simulink model "FLIGHT_Hexacopter_V2"  (R2025a)
settings: Solver=FixedStepDiscrete  StartTime=0.0  StopTime=inf  FixedStep=SampleTime_SAS  RelTol=1e-3  EnableMultiTasking=on
InitFcn:
  | Init_FLIGHT_Hexacopter
values from neighbouring files (symbols this model uses):
  d2r = pi/180    (= 0.0174532925199)    [Init_FLIGHT_Hexacopter.m]
  Kdrr = 0.004    [Init_FLIGHT_Hexacopter_fromNCMS.m]
  Kirr = 0.0    (= 0)    [Init_FLIGHT_Hexacopter_fromNCMS.m]
  Kpp = 3.3894    [Init_FLIGHT_Hexacopter_fromNCMS.m]
  Kpr = 3.3894    [Init_FLIGHT_Hexacopter_fromNCMS.m]
  Kprr = 0.1    [Init_FLIGHT_Hexacopter_fromNCMS.m]
  MAX_CONTROL_ANGLE_PITCH = 30*pi/180    (= 0.523598775598)    [Init_FLIGHT_Hexacopter.m]    (also in Init_FLIGHT_Hexacopter_fromNCMS.m = 0.349065850399)
  MAX_CONTROL_ANGLE_RATE_PITCH = 360*pi/180    (= 6.28318530718)    [Init_FLIGHT_Hexacopter.m]    (also in Init_FLIGHT_Hexacopter_fromNCMS.m)
  MAX_CONTROL_ANGLE_RATE_ROLL = 360*pi/180    (= 6.28318530718)    [Init_FLIGHT_Hexacopter.m]    (also in Init_FLIGHT_Hexacopter_fromNCMS.m)
  MAX_CONTROL_ANGLE_RATE_Y = 120*pi/180    (= 2.09439510239)    [Init_FLIGHT_Hexacopter.m]    (also in Init_FLIGHT_Hexacopter_fromNCMS.m)
  MAX_CONTROL_ANGLE_ROLL = 30*pi/180    (= 0.523598775598)    [Init_FLIGHT_Hexacopter.m]    (also in Init_FLIGHT_Hexacopter_fromNCMS.m = 0.349065850399)
  Nrr = 50    [Init_FLIGHT_Hexacopter_fromNCMS.m]
  PITCH_AUTHORITY = 1    [Init_FLIGHT_Hexacopter.m]
  ROLL_AUTHORITY = 1    [Init_FLIGHT_Hexacopter.m]
  SampleTime = 1/250    (= 0.004)    [Init_FLIGHT_Hexacopter.m]    (also in Init_FLIGHT_Hexacopter_fromNCMS.m = 0.01)
  SampleTime_SAS = 1/1000    (= 0.001)    [Init_FLIGHT_Hexacopter.m]
  YAW_AUTHORITY = 1    [Init_FLIGHT_Hexacopter.m]
undefined symbols (not defined in the file or in its folder): arguments, DiscIntNeverNeededParam, e_dot, event_sequence, fx, g1x, hx, id, integral_e, log_levels, MPC_Z_D, MPC_Z_I, MPC_Z_P, noutputs, omega, omega_dot, output, phi_cmd, phi_cmd_ddot, phi_cmd_dot, r, s, tau_roll, timestamp, w
libraries: px4Utilslib x65, simulink x21, px4uORBlib x12, slpidlib x9, cstblocks x5, simulink_extras x2, sharedtransform x1, px4Sensorslib x1, matrix_library x1, px4Peripheralslib x1
(part 2 of 3)

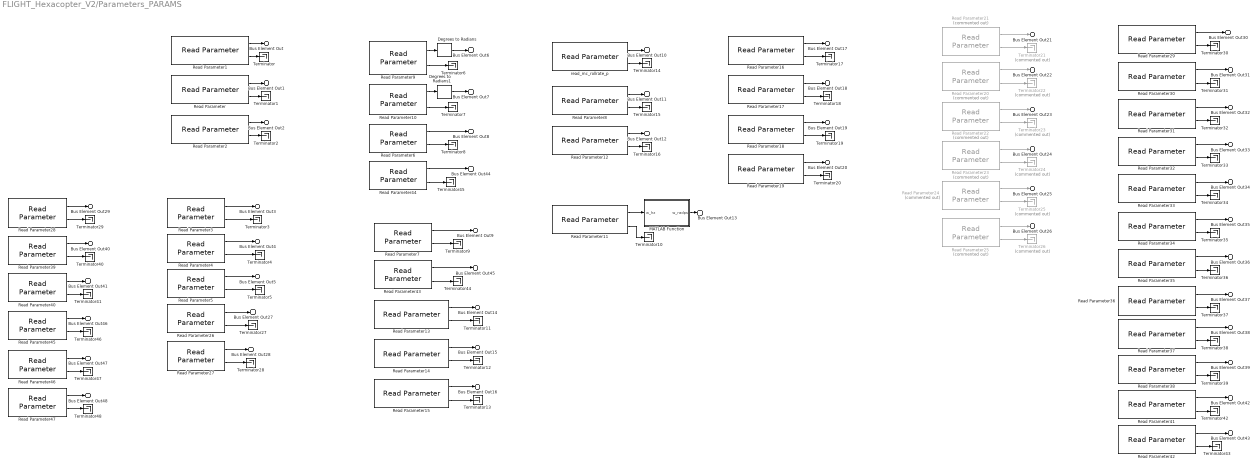
== system FLIGHT_Hexacopter_V2/Parameters_PARAMS ==
  Degrees to Radians : simulink_extras/Transformations/Degrees to Radians
  Degrees to Radians1 : simulink_extras/Transformations/Degrees to Radians
  MATLAB Function : MATLAB Function  TreatAsAtomicUnit=on
  Read Parameter : px4Utilslib/Read Parameter  ParameterName=DOUBLET_DT  DataType=FLOAT  SampleTime=SampleTime
  Read Parameter1 : px4Utilslib/Read Parameter  ParameterName=DOUBLET_PEAK_ANG  DataType=FLOAT  SampleTime=SampleTime
  Read Parameter10 : px4Utilslib/Read Parameter  ParameterName=MC_PITCHRATE_MAX  DataType=FLOAT  SampleTime=SampleTime
  Read Parameter11 : px4Utilslib/Read Parameter  ParameterName=IMU_DGYRO_CUTOFF  DataType=FLOAT  SampleTime=SampleTime
  Read Parameter12 : px4Utilslib/Read Parameter  ParameterName=MC_ROLLRATE_D  DataType=FLOAT  SampleTime=SampleTime
  Read Parameter13 : px4Utilslib/Read Parameter  ParameterName=MC_PITCHRATE_P  DataType=FLOAT  SampleTime=SampleTime
  Read Parameter14 : px4Utilslib/Read Parameter  ParameterName=MC_PITCHRATE_I  DataType=FLOAT  SampleTime=SampleTime
  Read Parameter15 : px4Utilslib/Read Parameter  ParameterName=MC_PITCHRATE_D  DataType=FLOAT  SampleTime=SampleTime
  Read Parameter16 : px4Utilslib/Read Parameter  ParameterName=MC_YAWRATE_P  DataType=FLOAT  SampleTime=SampleTime
  Read Parameter17 : px4Utilslib/Read Parameter  ParameterName=MC_YAWRATE_I  DataType=FLOAT  SampleTime=SampleTime
  Read Parameter18 : px4Utilslib/Read Parameter  ParameterName=MC_YAWRATE_D  DataType=FLOAT  SampleTime=SampleTime
  Read Parameter19 : px4Utilslib/Read Parameter  ParameterName=MC_YAWRATE_FF  DataType=FLOAT  SampleTime=SampleTime
  Read Parameter2 : px4Utilslib/Read Parameter  ParameterName=DOUBLET_AXIS  DataType=INT32  SampleTime=SampleTime
  Read Parameter20 : px4Utilslib/Read Parameter  Commented=on  ParameterName=FDD_M2_STATUS  DataType=INT32  SampleTime=SampleTime
  Read Parameter21 : px4Utilslib/Read Parameter  Commented=on  ParameterName=FDD_M1_STATUS  DataType=INT32  SampleTime=SampleTime
  Read Parameter22 : px4Utilslib/Read Parameter  Commented=on  ParameterName=FDD_M3_STATUS  DataType=INT32  SampleTime=SampleTime
  Read Parameter23 : px4Utilslib/Read Parameter  Commented=on  ParameterName=FDD_M4_STATUS  DataType=INT32  SampleTime=SampleTime
  Read Parameter24 : px4Utilslib/Read Parameter  Commented=on  ParameterName=FDD_M5_STATUS  DataType=INT32  SampleTime=SampleTime
  Read Parameter25 : px4Utilslib/Read Parameter  Commented=on  ParameterName=FDD_M6_STATUS  DataType=INT32  SampleTime=SampleTime
  Read Parameter26 : px4Utilslib/Read Parameter  ParameterName=MPC_THR_HOVER  DataType=FLOAT  SampleTime=SampleTime
  Read Parameter27 : px4Utilslib/Read Parameter  ParameterName=MPC_XY_P  DataType=FLOAT  SampleTime=SampleTime
  Read Parameter28 : px4Utilslib/Read Parameter  ParameterName=MPC_XY_VEL_P_ACC  DataType=FLOAT  SampleTime=SampleTime
  Read Parameter29 : px4Utilslib/Read Parameter  ParameterName=SMC_K_SS_P  DataType=FLOAT  SampleTime=SampleTime
  Read Parameter3 : px4Utilslib/Read Parameter  ParameterName=MPC_Z_VEL_P_ACC  DataType=FLOAT  SampleTime=SampleTime
  Read Parameter30 : px4Utilslib/Read Parameter  ParameterName=SMC_K_SS_I  DataType=FLOAT  SampleTime=SampleTime
  Read Parameter31 : px4Utilslib/Read Parameter  ParameterName=SMC_K_SS_D  DataType=FLOAT  SampleTime=SampleTime
  Read Parameter32 : px4Utilslib/Read Parameter  ParameterName=SMC_K_REACH_S  DataType=FLOAT  SampleTime=SampleTime
  Read Parameter33 : px4Utilslib/Read Parameter  ParameterName=SMC_K_REACH_P  DataType=FLOAT  SampleTime=SampleTime
  Read Parameter34 : px4Utilslib/Read Parameter  ParameterName=SMC_I_XX  DataType=FLOAT  SampleTime=SampleTime
  Read Parameter35 : px4Utilslib/Read Parameter  ParameterName=SMC_I_YY  DataType=FLOAT  SampleTime=SampleTime
  Read Parameter36 : px4Utilslib/Read Parameter  ParameterName=SMC_I_ZZ  DataType=FLOAT  SampleTime=SampleTime
  Read Parameter37 : px4Utilslib/Read Parameter  ParameterName=SMC_EPSILON  DataType=FLOAT  SampleTime=SampleTime
  Read Parameter38 : px4Utilslib/Read Parameter  ParameterName=SMC_LPF_CUTOFF  DataType=FLOAT  SampleTime=SampleTime
  Read Parameter39 : px4Utilslib/Read Parameter  ParameterName=MPC_Z_VEL_MAX_UP  DataType=FLOAT  SampleTime=SampleTime
  Read Parameter4 : px4Utilslib/Read Parameter  ParameterName=MPC_Z_VEL_I_ACC  DataType=FLOAT  SampleTime=SampleTime
  Read Parameter40 : px4Utilslib/Read Parameter  ParameterName=MPC_XY_VEL_MAX  DataType=FLOAT  SampleTime=SampleTime
  Read Parameter41 : px4Utilslib/Read Parameter  ParameterName=ST_SMC_LAMBDA  DataType=FLOAT  SampleTime=SampleTime
  Read Parameter42 : px4Utilslib/Read Parameter  ParameterName=ST_SMC_ETA  DataType=FLOAT  SampleTime=SampleTime
  Read Parameter43 : px4Utilslib/Read Parameter  ParameterName=MC_PITCH_I  DataType=FLOAT  SampleTime=SampleTime
  Read Parameter44 : px4Utilslib/Read Parameter  ParameterName=MC_ROLL_I  DataType=FLOAT  SampleTime=SampleTime
  Read Parameter45 : px4Utilslib/Read Parameter  ParameterName=MPC_XY_VEL_I_ACC  DataType=FLOAT  SampleTime=SampleTime
  Read Parameter46 : px4Utilslib/Read Parameter  ParameterName=MPC_XY_VEL_D_ACC  DataType=FLOAT  SampleTime=SampleTime
  Read Parameter47 : px4Utilslib/Read Parameter  ParameterName=MPC_WP_LENGTH  DataType=FLOAT  SampleTime=SampleTime
  Read Parameter5 : px4Utilslib/Read Parameter  ParameterName=MPC_Z_VEL_D_ACC  DataType=FLOAT  SampleTime=SampleTime
  Read Parameter6 : px4Utilslib/Read Parameter  ParameterName=MC_ROLL_P  DataType=FLOAT  SampleTime=SampleTime
  Read Parameter7 : px4Utilslib/Read Parameter  ParameterName=MC_PITCH_P  DataType=FLOAT  SampleTime=SampleTime
  Read Parameter8 : px4Utilslib/Read Parameter  ParameterName=MC_ROLLRATE_I  DataType=FLOAT  SampleTime=SampleTime
  Read Parameter9 : px4Utilslib/Read Parameter  ParameterName=MC_ROLLRATE_MAX  DataType=FLOAT  SampleTime=SampleTime
  Terminator{,1..20,27..48} (43 alike) : Terminator
  Terminator{21..26} (6 alike) : Terminator  Commented=on
  read_mc_rollrate_p : px4Utilslib/Read Parameter  ParameterName=MC_ROLLRATE_P  DataType=FLOAT  SampleTime=SampleTime
  Bus Element Out : Outport  PortName=PARAMS  Element=DOUBLET_PEAK_ANG
  Bus Element Out1 : Outport  PortName=PARAMS  Element=DOUBLET_DT
  Bus Element Out2 : Outport  PortName=PARAMS  Element=DOUBLET_AXIS
  Bus Element Out3 : Outport  PortName=PARAMS  Element=MPC_Z_VEL_P_ACC
  Bus Element Out4 : Outport  PortName=PARAMS  Element=MPC_Z_VEL_I_ACC
  Bus Element Out5 : Outport  PortName=PARAMS  Element=MPC_Z_VEL_D_ACC
  Bus Element Out6 : Outport  PortName=PARAMS  Element=MC_ROLLRATE_MAX
  Bus Element Out7 : Outport  PortName=PARAMS  Element=MC_PITCHRATE_MAX
  Bus Element Out8 : Outport  PortName=PARAMS  Element=MC_ROLL_P
  Bus Element Out9 : Outport  PortName=PARAMS  Element=MC_PITCH_P
  Bus Element Out10 : Outport  PortName=PARAMS  Element=MC_ROLLRATE_P
  Bus Element Out11 : Outport  PortName=PARAMS  Element=MC_ROLLRATE_I
  Bus Element Out12 : Outport  PortName=PARAMS  Element=MC_ROLLRATE_D
  Bus Element Out13 : Outport  PortName=PARAMS  Element=IMU_DGYRO_CUTOFF
  Bus Element Out14 : Outport  PortName=PARAMS  Element=MC_PITCHRATE_P
  Bus Element Out15 : Outport  PortName=PARAMS  Element=MC_PITCHRATE_I
  Bus Element Out16 : Outport  PortName=PARAMS  Element=MC_PITCHRATE_D
  Bus Element Out17 : Outport  PortName=PARAMS  Element=MC_YAWRATE_P
  Bus Element Out18 : Outport  PortName=PARAMS  Element=MC_YAWRATE_I
  Bus Element Out19 : Outport  PortName=PARAMS  Element=MC_YAWRATE_D
  Bus Element Out20 : Outport  PortName=PARAMS  Element=MC_YAWRATE_FF
  Bus Element Out21 : Outport  PortName=PARAMS  Element=FDD_M1_STATUS
  Bus Element Out22 : Outport  PortName=PARAMS  Element=FDD_M2_STATUS
  Bus Element Out23 : Outport  PortName=PARAMS  Element=FDD_M3_STATUS
  Bus Element Out24 : Outport  PortName=PARAMS  Element=FDD_M4_STATUS
  Bus Element Out25 : Outport  PortName=PARAMS  Element=FDD_M5_STATUS
  Bus Element Out26 : Outport  PortName=PARAMS  Element=FDD_M6_STATUS
  Bus Element Out27 : Outport  PortName=PARAMS  Element=MPC_THR_HOVER
  Bus Element Out28 : Outport  PortName=PARAMS  Element=MPC_XY_P
  Bus Element Out29 : Outport  PortName=PARAMS  Element=MPC_XY_VEL_P_ACC
  Bus Element Out30 : Outport  PortName=PARAMS  Element=K_SMC_P
  Bus Element Out31 : Outport  PortName=PARAMS  Element=K_SMC_I
  Bus Element Out32 : Outport  PortName=PARAMS  Element=K_SMC_D
  Bus Element Out33 : Outport  PortName=PARAMS  Element=K_REACH_S
  Bus Element Out34 : Outport  PortName=PARAMS  Element=K_REACH_P
  Bus Element Out35 : Outport  PortName=PARAMS  Element=I_XX
  Bus Element Out36 : Outport  PortName=PARAMS  Element=I_YY
  Bus Element Out37 : Outport  PortName=PARAMS  Element=I_ZZ
  Bus Element Out38 : Outport  PortName=PARAMS  Element=EPSILON
  Bus Element Out39 : Outport  PortName=PARAMS  Element=SMC_LPF_CUTOFF
  Bus Element Out40 : Outport  PortName=PARAMS  Element=MPC_Z_VEL_MAX_UP
  Bus Element Out41 : Outport  PortName=PARAMS  Element=MPC_XY_VEL_MAX
  Bus Element Out42 : Outport  PortName=PARAMS  Element=ST_SMC_LAMBDA
  Bus Element Out43 : Outport  PortName=PARAMS  Element=ST_SMC_ETA
  Bus Element Out44 : Outport  PortName=PARAMS  Element=MC_ROLL_I
  Bus Element Out45 : Outport  PortName=PARAMS  Element=MC_PITCH_I
  Bus Element Out46 : Outport  PortName=PARAMS  Element=MPC_XY_VEL_I_ACC
  Bus Element Out47 : Outport  PortName=PARAMS  Element=MPC_XY_VEL_D_ACC
  Bus Element Out48 : Outport  PortName=PARAMS  Element=MPC_WP_LENGTH
  wires:
  Read Parameter9/2 -> Terminator6/1
  Read Parameter10/1 -> Degrees to Radians1/1
  Read Parameter9/1 -> Degrees to Radians/1
  Read Parameter10/2 -> Terminator7/1
  Read Parameter7/1 -> Bus Element Out9/1
  Read Parameter7/2 -> Terminator9/1
  Read Parameter6/1 -> Bus Element Out8/1
  Read Parameter6/2 -> Terminator8/1
  Read Parameter11/2 -> Terminator10/1
  Read Parameter11/1 -> MATLAB Function/1(w_hz)
  Read Parameter1/1 -> Bus Element Out/1
  Read Parameter1/2 -> Terminator/1
  Read Parameter2/1 -> Bus Element Out2/1
  Read Parameter2/2 -> Terminator2/1
  Read Parameter/2 -> Terminator1/1
  Read Parameter/1 -> Bus Element Out1/1
  Read Parameter3/1 -> Bus Element Out3/1
  Read Parameter4/1 -> Bus Element Out4/1
  Read Parameter5/1 -> Bus Element Out5/1
  Read Parameter3/2 -> Terminator3/1
  Read Parameter4/2 -> Terminator4/1
  Read Parameter5/2 -> Terminator5/1
  Degrees to Radians1/1 -> Bus Element Out7/1
  Degrees to Radians/1 -> Bus Element Out6/1
  read_mc_rollrate_p/1 -> Bus Element Out10/1
  Read Parameter8/1 -> Bus Element Out11/1
  Read Parameter12/1 -> Bus Element Out12/1
  MATLAB Function/1(w_radps) -> Bus Element Out13/1
  Read Parameter13/1 -> Bus Element Out14/1
  Read Parameter14/1 -> Bus Element Out15/1
  Read Parameter15/1 -> Bus Element Out16/1
  Read Parameter13/2 -> Terminator11/1
  Read Parameter14/2 -> Terminator12/1
  Read Parameter15/2 -> Terminator13/1
  read_mc_rollrate_p/2 -> Terminator14/1
  Read Parameter8/2 -> Terminator15/1
  Read Parameter12/2 -> Terminator16/1
  Read Parameter16/1 -> Bus Element Out17/1
  Read Parameter17/1 -> Bus Element Out18/1
  Read Parameter18/1 -> Bus Element Out19/1
  Read Parameter19/1 -> Bus Element Out20/1
  Read Parameter16/2 -> Terminator17/1
  Read Parameter17/2 -> Terminator18/1
  Read Parameter18/2 -> Terminator19/1
  Read Parameter19/2 -> Terminator20/1
  Read Parameter21/1 -> Bus Element Out21/1
  Read Parameter20/1 -> Bus Element Out22/1
  Read Parameter22/1 -> Bus Element Out23/1
  Read Parameter23/1 -> Bus Element Out24/1
  Read Parameter24/1 -> Bus Element Out25/1
  Read Parameter25/1 -> Bus Element Out26/1
  Read Parameter21/2 -> Terminator21/1
  Read Parameter20/2 -> Terminator22/1
  Read Parameter22/2 -> Terminator23/1
  Read Parameter23/2 -> Terminator24/1
  Read Parameter24/2 -> Terminator25/1
  Read Parameter25/2 -> Terminator26/1
  Read Parameter26/1 -> Bus Element Out27/1
  Read Parameter26/2 -> Terminator27/1
  Read Parameter27/1 -> Bus Element Out28/1
  Read Parameter27/2 -> Terminator28/1
  Read Parameter28/1 -> Bus Element Out29/1
  Read Parameter28/2 -> Terminator29/1
  Read Parameter32/1 -> Bus Element Out33/1
  Read Parameter33/2 -> Terminator34/1
  Read Parameter31/2 -> Terminator32/1
  Read Parameter33/1 -> Bus Element Out34/1
  Read Parameter29/1 -> Bus Element Out30/1
  Read Parameter30/2 -> Terminator31/1
  Read Parameter30/1 -> Bus Element Out31/1
  Read Parameter32/2 -> Terminator33/1
  Read Parameter31/1 -> Bus Element Out32/1
  Read Parameter29/2 -> Terminator30/1
  Read Parameter34/1 -> Bus Element Out35/1
  Read Parameter34/2 -> Terminator35/1
  Read Parameter35/1 -> Bus Element Out36/1
  Read Parameter35/2 -> Terminator36/1
  Read Parameter36/1 -> Bus Element Out37/1
  Read Parameter36/2 -> Terminator37/1
  Read Parameter37/1 -> Bus Element Out38/1
  Read Parameter37/2 -> Terminator38/1
  Read Parameter38/1 -> Bus Element Out39/1
  Read Parameter38/2 -> Terminator39/1
  Read Parameter39/2 -> Terminator40/1
  Read Parameter39/1 -> Bus Element Out40/1
  Read Parameter40/1 -> Bus Element Out41/1
  Read Parameter40/2 -> Terminator41/1
  Read Parameter41/1 -> Bus Element Out42/1
  Read Parameter41/2 -> Terminator42/1
  Read Parameter42/1 -> Bus Element Out43/1
  Read Parameter42/2 -> Terminator43/1
  Read Parameter43/1 -> Bus Element Out45/1
  Read Parameter43/2 -> Terminator44/1
  Read Parameter44/1 -> Bus Element Out44/1
  Read Parameter44/2 -> Terminator45/1
  Read Parameter45/1 -> Bus Element Out46/1
  Read Parameter46/1 -> Bus Element Out47/1
  Read Parameter45/2 -> Terminator46/1
  Read Parameter46/2 -> Terminator47/1
  Read Parameter47/1 -> Bus Element Out48/1
  Read Parameter47/2 -> Terminator48/1

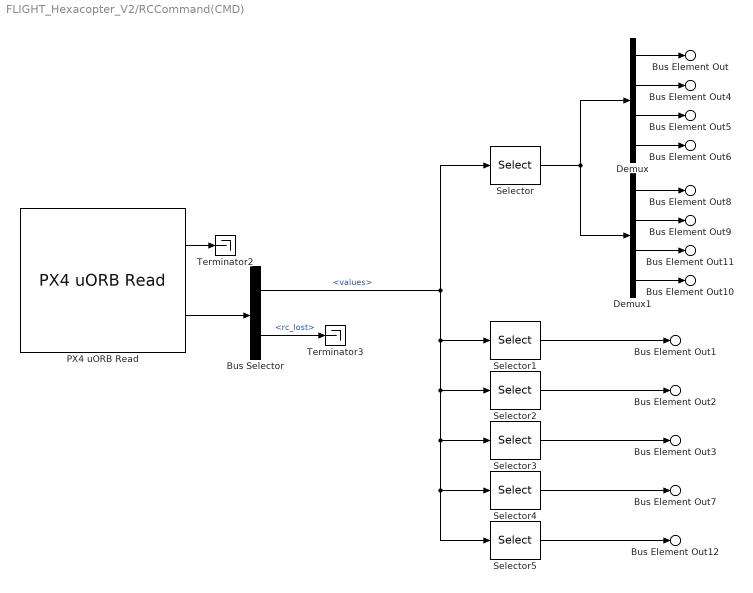
== system FLIGHT_Hexacopter_V2/RCCommand(CMD) ==
  Bus Selector : BusSelector  OutputSignals=values,rc_lost
  Demux : Demux
  Demux1 : Demux
  PX4 uORB Read : px4uORBlib/PX4 uORB Read  uORBTopic=InputRc  selectInstance=InputRc  SampleTime=SampleTime  BlockingMode=off  BlockTimeout=1e-3
  Selector : Selector  InputPortWidth=18  IndexOptions=Index vector (dialog)  Indices=[1 2 4 3]  OutputSizes=1
  Selector1 : Selector  InputPortWidth=18  IndexOptions=Index vector (dialog)  Indices=[6]  OutputSizes=1
  Selector2 : Selector  InputPortWidth=18  IndexOptions=Index vector (dialog)  Indices=7  OutputSizes=1
  Selector3 : Selector  InputPortWidth=18  IndexOptions=Index vector (dialog)  Indices=8  OutputSizes=1
  Selector4 : Selector  InputPortWidth=18  IndexOptions=Index vector (dialog)  Indices=10  OutputSizes=1
  Selector5 : Selector  InputPortWidth=18  IndexOptions=Index vector (dialog)  Indices=11  OutputSizes=1
  Terminator2 : Terminator
  Terminator3 : Terminator
  Bus Element Out : Outport  PortName=CMD  Element=rc_mode2_roll
  Bus Element Out1 : Outport  PortName=CMD  Element=rc_mode
  Bus Element Out2 : Outport  PortName=CMD  Element=rc_doublet
  Bus Element Out3 : Outport  PortName=CMD  Element=rc_inject_failure
  Bus Element Out4 : Outport  PortName=CMD  Element=rc_mode2_pitch
  Bus Element Out5 : Outport  PortName=CMD  Element=rc_mode2_yaw
  Bus Element Out6 : Outport  PortName=CMD  Element=rc_mode2_throttle
  Bus Element Out7 : Outport  PortName=CMD  Element=rc_ctrl_switch
  Bus Element Out8 : Outport  PortName=CMD  Element=rc_mode1_roll
  Bus Element Out9 : Outport  PortName=CMD  Element=rc_mode1_throttle
  Bus Element Out10 : Outport  PortName=CMD  Element=rc_mode1_pitch
  Bus Element Out11 : Outport  PortName=CMD  Element=rc_mode1_yaw
  Bus Element Out12 : Outport  PortName=CMD  Element=rc_ap_sw
  wires:
  Selector/1 -> Demux1/1, Demux/1
  PX4 uORB Read/2 -> Bus Selector/1
  Bus Selector/2 -> Terminator3/1  "<rc_lost>"
  Selector1/1 -> Bus Element Out1/1
  Bus Selector/1 -> Selector5/1, Selector4/1, Selector3/1, Selector2/1, Selector1/1, Selector/1  "<values>"
  PX4 uORB Read/1 -> Terminator2/1
  Demux/1 -> Bus Element Out/1
  Demux/2 -> Bus Element Out4/1
  Demux/3 -> Bus Element Out5/1
  Demux/4 -> Bus Element Out6/1
  Selector2/1 -> Bus Element Out2/1
  Selector3/1 -> Bus Element Out3/1
  Selector4/1 -> Bus Element Out7/1
  Demux1/1 -> Bus Element Out8/1
  Demux1/2 -> Bus Element Out9/1
  Demux1/3 -> Bus Element Out11/1
  Demux1/4 -> Bus Element Out10/1
  Selector5/1 -> Bus Element Out12/1

== system FLIGHT_Hexacopter_V2/Read_uORB(1000hz)_SENSORS1000 ==
  Bus Selector2 : BusSelector  OutputSignals=xyz,xyz_derivative
  Demux : Demux  Outputs=3
  Demux1 : Demux  Outputs=3
  PX4 uORB Read1 : px4uORBlib/PX4 uORB Read  uORBTopic=VehicleAngularVelocity  selectInstance=vehicle_angular_velocity  SampleTime=SampleTime_SAS  BlockingMode=off  BlockTimeout=1e-3
  Terminator1 : Terminator
  Bus Element Out : Outport  PortName=SENSORS1000  Element=P
  Bus Element Out1 : Outport  PortName=SENSORS1000  Element=Q
  Bus Element Out2 : Outport  PortName=SENSORS1000  Element=R
  Bus Element Out3 : Outport  PortName=SENSORS1000  Element=P_dot
  Bus Element Out4 : Outport  PortName=SENSORS1000  Element=Q_dot
  Bus Element Out5 : Outport  PortName=SENSORS1000  Element=R_dot
  wires:
  Bus Selector2/1 -> Demux/1  "<xyz>"
  PX4 uORB Read1/1 -> Terminator1/1
  Bus Selector2/2 -> Demux1/1  "<xyz_derivative>"
  PX4 uORB Read1/2 -> Bus Selector2/1
  Demux/1 -> Bus Element Out/1
  Demux/2 -> Bus Element Out1/1
  Demux/3 -> Bus Element Out2/1
  Demux1/1 -> Bus Element Out3/1
  Demux1/2 -> Bus Element Out4/1
  Demux1/3 -> Bus Element Out5/1

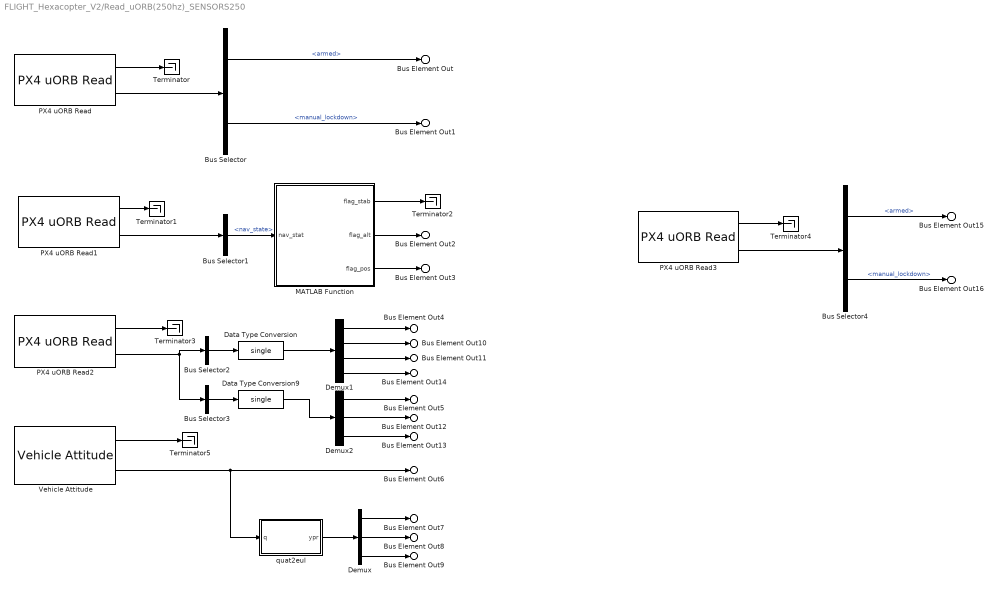
== system FLIGHT_Hexacopter_V2/Read_uORB(250hz)_SENSORS250 ==
  Bus Selector : BusSelector  OutputSignals=armed,manual_lockdown
  Bus Selector1 : BusSelector  OutputSignals=nav_state
  Bus Selector2 : BusSelector  OutputSignals=x,y,z,heading  OutputAsBus=on
  Bus Selector3 : BusSelector  OutputSignals=vx,vy,vz  OutputAsBus=on
  Bus Selector4 : BusSelector  OutputSignals=armed,manual_lockdown
  Data Type Conversion : DataTypeConversion  OutDataTypeStr=single  SaturateOnIntegerOverflow=off  RndMeth=Floor
  Data Type Conversion9 : DataTypeConversion  OutDataTypeStr=single  SaturateOnIntegerOverflow=off  RndMeth=Floor
  Demux : Demux  Outputs=3
  Demux1 : Demux
  Demux2 : Demux  Outputs=3
  MATLAB Function : MATLAB Function  TreatAsAtomicUnit=on
  PX4 uORB Read : px4uORBlib/PX4 uORB Read  uORBTopic=ActuatorArmed  selectInstance=ActuatorArmed  SampleTime=SampleTime  BlockingMode=off  BlockTimeout=1e-3
  PX4 uORB Read1 : px4uORBlib/PX4 uORB Read  uORBTopic=VehicleStatus  selectInstance=VehicleStatus  SampleTime=SampleTime  BlockingMode=off  BlockTimeout=1e-3
  PX4 uORB Read2 : px4uORBlib/PX4 uORB Read  uORBTopic=VehicleLocalPosition  selectInstance=vehicle_local_position  SampleTime=SampleTime  BlockingMode=off  BlockTimeout=1e-3
  PX4 uORB Read3 : px4uORBlib/PX4 uORB Read  uORBTopic=ActuatorArmed  selectInstance=ActuatorArmed  SampleTime=SampleTime  BlockingMode=off  BlockTimeout=1e-3
  Terminator{,1..5} (6 alike) : Terminator
  Vehicle Attitude : px4Sensorslib/Vehicle Attitude  rollRate=off  pitchRate=off  yawRate=off  quaternion=on  uorbTimeStamp=off  BlockingMode=off  BlockTimeout=0.001  sampleTime=SampleTime
  quat2eul : MATLAB Function  TreatAsAtomicUnit=on
  Bus Element Out : Outport  PortName=SENSORS250  Element=VehicleStatus_armed
  Bus Element Out1 : Outport  PortName=SENSORS250  Element=VehicleStatus_emergency_kill
  Bus Element Out2 : Outport  PortName=SENSORS250  Element=VehicleStatus_flag_altitude_mode
  Bus Element Out3 : Outport  PortName=SENSORS250  Element=VehicleStatus_flag_position_mode
  Bus Element Out4 : Outport  PortName=SENSORS250  Element=X
  Bus Element Out5 : Outport  PortName=SENSORS250  Element=U
  Bus Element Out6 : Outport  PortName=SENSORS250  Element=State_quaternion
  Bus Element Out7 : Outport  PortName=SENSORS250  Element=Psi
  Bus Element Out8 : Outport  PortName=SENSORS250  Element=Theta
  Bus Element Out9 : Outport  PortName=SENSORS250  Element=Phi
  Bus Element Out12 : Outport  PortName=SENSORS250  Element=V
  Bus Element Out13 : Outport  PortName=SENSORS250  Element=W
  Bus Element Out10 : Outport  PortName=SENSORS250  Element=Y
  Bus Element Out11 : Outport  PortName=SENSORS250  Element=Z
  Bus Element Out14 : Outport  PortName=SENSORS250  Element=Heading
  Bus Element Out15 : Outport  PortName=SENSORS250  Element=VehicleStatus_flag_armed
  Bus Element Out16 : Outport  PortName=SENSORS250  Element=VehicleStatus_flag_kill
  wires:
  Bus Selector/2 -> Bus Element Out1/1  "<manual_lockdown>"
  Bus Selector/1 -> Bus Element Out/1  "<armed>"
  PX4 uORB Read/1 -> Terminator/1
  PX4 uORB Read/2 -> Bus Selector/1
  PX4 uORB Read1/1 -> Terminator1/1
  PX4 uORB Read1/2 -> Bus Selector1/1
  MATLAB Function/3(flag_pos) -> Bus Element Out3/1
  Bus Selector1/1 -> MATLAB Function/1(nav_stat)  "<nav_state>"
  MATLAB Function/2(flag_alt) -> Bus Element Out2/1
  MATLAB Function/1(flag_stab) -> Terminator2/1
  Bus Selector3/1 -> Data Type Conversion9/1
  PX4 uORB Read2/1 -> Terminator3/1
  Bus Selector2/1 -> Data Type Conversion/1
  Vehicle Attitude/1 -> Terminator5/1
  PX4 uORB Read2/2 -> Bus Selector3/1, Bus Selector2/1
  Vehicle Attitude/2 -> quat2eul/1(q), Bus Element Out6/1
  quat2eul/1(ypr) -> Demux/1
  Demux/1 -> Bus Element Out7/1
  Demux/2 -> Bus Element Out8/1
  Demux/3 -> Bus Element Out9/1
  Data Type Conversion/1 -> Demux1/1
  Demux1/1 -> Bus Element Out4/1
  Demux1/2 -> Bus Element Out10/1
  Demux1/3 -> Bus Element Out11/1
  Data Type Conversion9/1 -> Demux2/1
  Demux2/1 -> Bus Element Out5/1
  Demux2/2 -> Bus Element Out12/1
  Demux2/3 -> Bus Element Out13/1
  Demux1/4 -> Bus Element Out14/1
  PX4 uORB Read3/2 -> Bus Selector4/1
  PX4 uORB Read3/1 -> Terminator4/1
  Bus Selector4/2 -> Bus Element Out16/1  "<manual_lockdown>"
  Bus Selector4/1 -> Bus Element Out15/1  "<armed>"

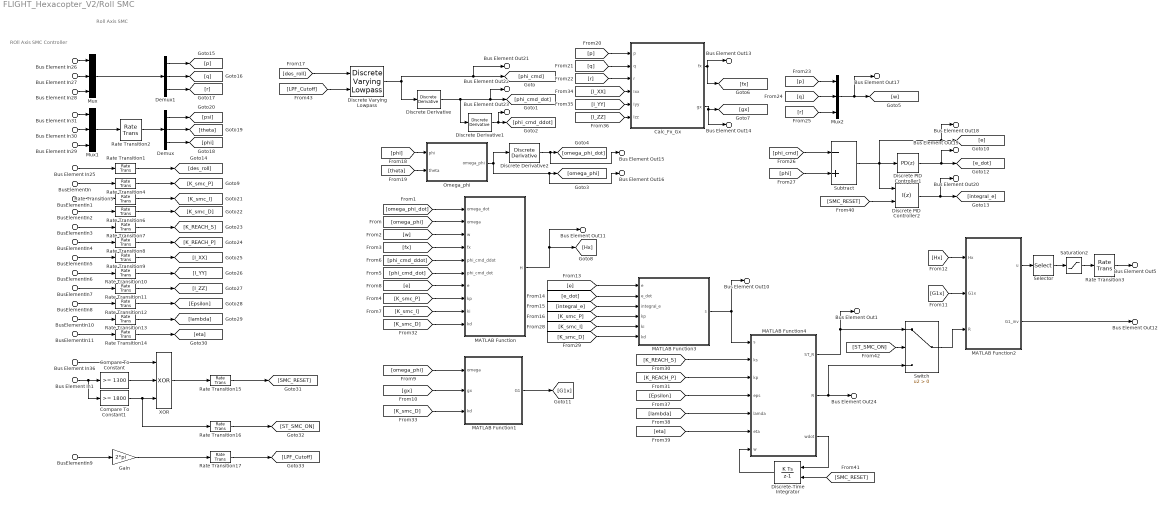
== system FLIGHT_Hexacopter_V2/Roll SMC ==
  note: Roll Axis SMC
  note: ROll Axis SMC Controller
  Bus Element In25 : Inport  PortName=OFP  Element=des_roll
  BusElementIn : Inport  Port=2  PortName=PARAMS  Element=K_SMC_P
  BusElementIn1 : Inport  Port=2  PortName=PARAMS  Element=K_SMC_I
  BusElementIn2 : Inport  Port=2  PortName=PARAMS  Element=K_SMC_D
  BusElementIn3 : Inport  Port=2  PortName=PARAMS  Element=K_REACH_S
  BusElementIn4 : Inport  Port=2  PortName=PARAMS  Element=K_REACH_P
  BusElementIn5 : Inport  Port=2  PortName=PARAMS  Element=I_XX
  BusElementIn6 : Inport  Port=2  PortName=PARAMS  Element=I_YY
  BusElementIn7 : Inport  Port=2  PortName=PARAMS  Element=I_ZZ
  BusElementIn8 : Inport  Port=2  PortName=PARAMS  Element=EPSILON
  BusElementIn9 : Inport  Port=2  PortName=PARAMS  Element=SMC_LPF_CUTOFF
  BusElementIn10 : Inport  Port=2  PortName=PARAMS  Element=ST_SMC_LAMBDA
  BusElementIn11 : Inport  Port=2  PortName=PARAMS  Element=ST_SMC_ETA
  Bus Element In29 : Inport  Port=3  PortName=SENSORS250  Element=Phi
  Bus Element In30 : Inport  Port=3  PortName=SENSORS250  Element=Theta
  Bus Element In31 : Inport  Port=3  PortName=SENSORS250  Element=Psi
  Bus Element In36 : Inport  Port=3  PortName=SENSORS250  Element=VehicleStatus_flag_armed
  Bus Element In26 : Inport  Port=4  PortName=SENSORS1000  Element=P
  Bus Element In27 : Inport  Port=4  PortName=SENSORS1000  Element=Q
  Bus Element In28 : Inport  Port=4  PortName=SENSORS1000  Element=R
  Bus Element In1 : Inport  Port=5  PortName=CMD  Element=rc_ctrl_switch
  Calc_Fx_Gx : Subsystem
  Compare To Constant : simulink/Logic and Bit Operations/Compare To Constant  relop=>=  const=1300  OutDataTypeStr=boolean
  Compare To Constant1 : simulink/Logic and Bit Operations/Compare To Constant  relop=>=  const=1800  OutDataTypeStr=boolean
  Demux : Demux  Outputs=3
  Demux1 : Demux  Outputs=3
  Discrete Derivative : simulink/Discrete/Discrete Derivative  gainval=1.0  ICPrevScaledInput=0.0  OutMin=[]  OutMax=[]  OutDataType=fixdt(1, 16)  OutScaling=2^-10  DoSatur=off
  Discrete Derivative1 : simulink/Discrete/Discrete Derivative  gainval=1.0  ICPrevScaledInput=0.0  OutMin=[]  OutMax=[]  OutDataType=fixdt(1, 16)  OutScaling=2^-10  DoSatur=off
  Discrete Derivative2 : simulink/Discrete/Discrete Derivative  gainval=1.0  ICPrevScaledInput=0.0  OutMin=[]  OutMax=[]  OutDataType=fixdt(1, 16)  OutScaling=2^-10  DoSatur=off
  Discrete PID Controller1 : slpidlib/PID Controller  Controller=PD  Form=Parallel  TimeDomain=Discrete-time  UseExternalTs=off  SampleTime=SampleTime_SAS  IntegratorMethod=Forward Euler  FilterMethod=Forward Euler  ControllerParametersSource=internal  P=0  I=1  UseKiTs=off  D=1  UseExternalDerivativeSource=off  N=100  UseFilter=on  TunerSelectOption=Transfer Function Based (PID Tuner App)  InitialConditionSource=internal  InitialConditionForIntegrator=0  InitialConditionForFilter=0  DifferentiatorICPrevScaledInput=0  ExternalReset=none  TrackingMode=off  Kt=1  LimitOutput=off  SatLimitsSource=internal  UpperSaturationLimit=inf  LowerSaturationLimit=-inf  LinearizeAsGain=off  AntiWindupMode=none  Kb=1  LimitIntegrator=off  UpperIntegratorSaturationLimit=inf  LowerIntegratorSaturationLimit=-inf  POutMin=[]  POutMax=[]  IOutMin=[]  IOutMax=[]  DOutMin=[]  DOutMax=[]  NOutMin=[]  NOutMax=[]  SumOutMin=[]  SumOutMax=[]  SaturationOutMin=[]  SaturationOutMax=[]  PParamMin=[]  PParamMax=[]  IParamMin=[]  IParamMax=[]  DParamMin=[]  DParamMax=[]  NParamMin=[]  NParamMax=[]  KbParamMin=[]  KbParamMax=[]  KtParamMin=[]  KtParamMax=[]  KbOutMin=[]  KbOutMax=[]  KtOutMin=[]  KtOutMax=[]  IntegratorOutMin=[]  IntegratorOutMax=[]  FilterOutMin=[]  FilterOutMax=[]  SumI1OutMin=[]  SumI1OutMax=[]  SumI2OutMin=[]  SumI2OutMax=[]  SumI3OutMin=[]  SumI3OutMax=[]  SumI4OutMin=[]  SumI4OutMax=[]  SumDOutMin=[]  SumDOutMax=[]  DifferentiatorOutMin=[]  DifferentiatorOutMax=[]  FilterDiffOutCoefMin=[]  FilterDiffOutCoefMax=[]  ReciprocalOutMin=[]  ReciprocalOutMax=[]  SumDenOutMin=[]  SumDenOutMax=[]  SumNumOutMin=[]  SumNumOutMax=[]  DivideOutMin=[]  DivideOutMax=[]  UdiffTsProdOutMin=[]  UdiffTsProdOutMax=[]  NTsProdOutMin=[]  NTsProdOutMax=[]  UintegralTsProdOutMin=[]  UintegralTsProdOutMax=[]  UngainTsProdOutMin=[]  UngainTsProdOutMax=[]  ClampingZeroOutDataTypeStr=Inherit: Inherit via back propagation  ClampingZeroOutMin=[]  ClampingZeroOutMax=[]  FilterDenConstantOutDataTypeStr=Inherit: Inherit via back propagation  FilterDenConstantOutMin=[]  FilterDenConstantOutMax=[]  PCopyOutDataTypeStr=Inherit: Inherit via back propagation  PCopyOutMin=[]  PCopyOutMax=[]  NCopyOutDataTypeStr=Inherit: Inherit via back propagation  NCopyOutMin=[]  NCopyOutMax=[]  IntegratorContinuousStateAttributes=''  IntegratorStateMustResolveToSignalObject=off  IntegratorRTWStateStorageClass=Auto  FilterContinuousStateAttributes=''  FilterStateMustResolveToSignalObject=off  FilterRTWStateStorageClass=Auto  ParallelPVariant=InternalParameters  IdealPVariant=Disabled  IVariant=Disabled  DVariant=InternalParameters  IntegratorVariant=Disabled  SatVariant=Disabled  AWVariant=Disabled  PCopyVariant=Disabled  TRVariant=Disabled  FdbkBlocksVariant=Forward  IdealPFdbkVariant=Disabled  SatFdbkVariant=Disabled  DerivativeFilterVariant=ForwardEulerFilter  NVariant=InternalParameters  NCopyVariant=Disabled  FilterICVariant=InternalICsFilter  IntegratorICVariant=Disabled  ExternalResetVariant=Disabled  TRSumVariant=Passthrough  SumFdbkVariant=Disabled  SumVariant=Sum_PD  TsampFilterVariant=InternalTs  TsampNgainVariant=Passthrough  TsampIntegralVariant=Disabled_SignalSpec  ExternalSaturationOutDataTypeStr=Inherit: Same as second input  DerivativeSourceVariant=ErrorSignal  PreIntVariant=InternalPreInt
      settings: LibrarySourceBlock=simulink/Discrete/Discrete PID Controller
  Discrete PID Controller2 : slpidlib/PID Controller  Controller=I  Form=Parallel  TimeDomain=Discrete-time  UseExternalTs=off  SampleTime=SampleTime_SAS  IntegratorMethod=Forward Euler  FilterMethod=Forward Euler  ControllerParametersSource=internal  P=1  I=1  UseKiTs=off  D=0  UseExternalDerivativeSource=off  N=100  UseFilter=on  TunerSelectOption=Transfer Function Based (PID Tuner App)  InitialConditionSource=internal  InitialConditionForIntegrator=0  InitialConditionForFilter=0  DifferentiatorICPrevScaledInput=0  ExternalReset=either  TrackingMode=off  Kt=1  LimitOutput=off  SatLimitsSource=internal  UpperSaturationLimit=inf  LowerSaturationLimit=-inf  LinearizeAsGain=off  AntiWindupMode=none  Kb=1  LimitIntegrator=off  UpperIntegratorSaturationLimit=inf  LowerIntegratorSaturationLimit=-inf  POutMin=[]  POutMax=[]  IOutMin=[]  IOutMax=[]  DOutMin=[]  DOutMax=[]  NOutMin=[]  NOutMax=[]  SumOutMin=[]  SumOutMax=[]  SaturationOutMin=[]  SaturationOutMax=[]  PParamMin=[]  PParamMax=[]  IParamMin=[]  IParamMax=[]  DParamMin=[]  DParamMax=[]  NParamMin=[]  NParamMax=[]  KbParamMin=[]  KbParamMax=[]  KtParamMin=[]  KtParamMax=[]  KbOutMin=[]  KbOutMax=[]  KtOutMin=[]  KtOutMax=[]  IntegratorOutMin=[]  IntegratorOutMax=[]  FilterOutMin=[]  FilterOutMax=[]  SumI1OutMin=[]  SumI1OutMax=[]  SumI2OutMin=[]  SumI2OutMax=[]  SumI3OutMin=[]  SumI3OutMax=[]  SumI4OutMin=[]  SumI4OutMax=[]  SumDOutMin=[]  SumDOutMax=[]  DifferentiatorOutMin=[]  DifferentiatorOutMax=[]  FilterDiffOutCoefMin=[]  FilterDiffOutCoefMax=[]  ReciprocalOutMin=[]  ReciprocalOutMax=[]  SumDenOutMin=[]  SumDenOutMax=[]  SumNumOutMin=[]  SumNumOutMax=[]  DivideOutMin=[]  DivideOutMax=[]  UdiffTsProdOutMin=[]  UdiffTsProdOutMax=[]  NTsProdOutMin=[]  NTsProdOutMax=[]  UintegralTsProdOutMin=[]  UintegralTsProdOutMax=[]  UngainTsProdOutMin=[]  UngainTsProdOutMax=[]  ClampingZeroOutDataTypeStr=Inherit: Inherit via back propagation  ClampingZeroOutMin=[]  ClampingZeroOutMax=[]  FilterDenConstantOutDataTypeStr=Inherit: Inherit via back propagation  FilterDenConstantOutMin=[]  FilterDenConstantOutMax=[]  PCopyOutDataTypeStr=Inherit: Inherit via back propagation  PCopyOutMin=[]  PCopyOutMax=[]  NCopyOutDataTypeStr=Inherit: Inherit via back propagation  NCopyOutMin=[]  NCopyOutMax=[]  IntegratorContinuousStateAttributes=''  IntegratorStateMustResolveToSignalObject=off  IntegratorRTWStateStorageClass=Auto  FilterContinuousStateAttributes=''  FilterStateMustResolveToSignalObject=off  FilterRTWStateStorageClass=Auto  ParallelPVariant=Disabled  IdealPVariant=Disabled  IVariant=InternalParameters  DVariant=Disabled  IntegratorVariant=Discrete  SatVariant=Disabled  AWVariant=Passthrough  PCopyVariant=Disabled  TRVariant=Disabled  FdbkBlocksVariant=Forward  IdealPFdbkVariant=Disabled  SatFdbkVariant=Disabled  DerivativeFilterVariant=Disabled  NVariant=Disabled  NCopyVariant=Disabled_SignalSpec  FilterICVariant=Disabled  IntegratorICVariant=InternalICs  ExternalResetVariant=ExternalReset  TRSumVariant=Passthrough  SumFdbkVariant=Disabled  SumVariant=Passthrough_I  TsampFilterVariant=InternalTs  TsampNgainVariant=Passthrough  TsampIntegralVariant=Disabled_SignalSpec  ExternalSaturationOutDataTypeStr=Inherit: Same as second input  DerivativeSourceVariant=Disabled  PreIntVariant=InternalPreInt
      settings: LibrarySourceBlock=simulink/Discrete/Discrete PID Controller
  Discrete Varying Lowpass : cstblocks/Linear Parameter Varying/Discrete Varying Lowpass  N=1  w0=0  Ts=SampleTime_SAS
  Discrete-Time Integrator : DiscreteIntegrator  ExternalReset=either  SampleTime=SampleTime_SAS  ICPrevOutput=DiscIntNeverNeededParam  ICPrevScaledInput=DiscIntNeverNeededParam
  Gain : Gain  Gain=2*pi
  MATLAB Function : MATLAB Function  TreatAsAtomicUnit=on
  MATLAB Function1 : MATLAB Function  TreatAsAtomicUnit=on
  MATLAB Function2 : MATLAB Function  TreatAsAtomicUnit=on
  MATLAB Function3 : MATLAB Function  TreatAsAtomicUnit=on
  MATLAB Function4 : MATLAB Function  TreatAsAtomicUnit=on
  Mux : Mux  Inputs=3
  Mux1 : Mux  Inputs=3
  Mux2 : Mux  Inputs=3
  Omega_phi : MATLAB Function  TreatAsAtomicUnit=on
  Rate Transition{1..17} (17 alike) : RateTransition  OutPortSampleTime=SampleTime_SAS
  Saturation2 : Saturate  UpperLimit=2  LowerLimit=-2
  Selector : Selector  InputPortWidth=3  IndexOptions=Index vector (dialog)  Indices=1  OutputSizes=1
  Subtract : Sum  Inputs=-+
  Switch : Switch  Criteria=u2 > Threshold  SaturateOnIntegerOverflow=off  InputSameDT=off
  XOR : Logic  Operator=XOR  Inputs=3  AllPortsSameDT=off  OutDataTypeStr=boolean
  Bus Element Out5 : Outport  PortName=SMC  Element=tau_roll
  Bus Element Out10 : Outport  PortName=SMC  Element=s
  Bus Element Out11 : Outport  PortName=SMC  Element=hx
  Bus Element Out12 : Outport  PortName=SMC  Element=g1x_inv
  Bus Element Out13 : Outport  PortName=SMC  Element=fx
  Bus Element Out14 : Outport  PortName=SMC  Element=gx
  Bus Element Out15 : Outport  PortName=SMC  Element=omega_phi_dot
  Bus Element Out16 : Outport  PortName=SMC  Element=omega_phi
  Bus Element Out17 : Outport  PortName=SMC  Element=w
  Bus Element Out18 : Outport  PortName=SMC  Element=e
  Bus Element Out19 : Outport  PortName=SMC  Element=e_dot
  Bus Element Out20 : Outport  PortName=SMC  Element=integral_e
  Bus Element Out21 : Outport  PortName=SMC  Element=phi_cmd
  Bus Element Out22 : Outport  PortName=SMC  Element=phi_cmd_dot
  Bus Element Out23 : Outport  PortName=SMC  Element=phi_cmd_ddot
  Bus Element Out24 : Outport  PortName=SMC  Element=r
  Bus Element Out1 : Outport  PortName=SMC  Element=st_r
  wires:
  [K_smc_I] -> MATLAB Function/9(ki)
  Bus Element In30/1 -> Mux1/2
  [omega_phi_dot] -> MATLAB Function/1(omega_dot)
  Demux1/1 -> [p]
  [K_smc_P] -> MATLAB Function/8(kp)
  MATLAB Function2/1(u) -> Selector/1
  Mux2/1 -> Bus Element Out17/1, [w]
  [q] -> Mux2/2
  [e_dot] -> MATLAB Function3/2(e_dot)
  [phi] -> Subtract/2
  BusElementIn3/1 -> Rate Transition7/1
  [r] -> Calc_Fx_Gx/3(r)
  Saturation2/1 -> Rate Transition3/1
  Bus Element In28/1 -> Mux/3
  [phi_cmd_dot] -> MATLAB Function/6(phi_cmd_dot)
  Bus Element In27/1 -> Mux/2
  Discrete PID Controller1/1 -> Bus Element Out19/1, [e_dot]
  [theta] -> Omega_phi/2(theta)
  Demux/2 -> [theta]
  [des_roll] -> Discrete Varying Lowpass/1
  Omega_phi/1(omega_phi) -> Discrete Derivative2/1, Bus Element Out16/1, [omega_phi]
  BusElementIn4/1 -> Rate Transition8/1
  MATLAB Function1/1(G1) -> [G1x]
  Calc_Fx_Gx/2(gx) -> Bus Element Out14/1, [gx]
  Discrete Derivative1/1 -> Bus Element Out23/1, [phi_cmd_ddot]
  Subtract/1 -> Discrete PID Controller2/1, Discrete PID Controller1/1, Bus Element Out18/1, [e]
  Discrete PID Controller2/1 -> Bus Element Out20/1, [integral_e]
  [K_smc_D] -> MATLAB Function/10(kd)
  Selector/1 -> Saturation2/1
  Discrete Derivative2/1 -> Bus Element Out15/1, [omega_phi_dot]
  MATLAB Function4/2(R) -> Switch/3, Bus Element Out24/1
  [p] -> Mux2/1
  [omega_phi] -> MATLAB Function/2(omega)
  [phi_cmd_ddot] -> MATLAB Function/5(phi_cmd_ddot)
  [gx] -> MATLAB Function1/2(gx)
  [K_REACH_S] -> MATLAB Function4/2(ks)
  [r] -> Mux2/3
  BusElementIn1/1 -> Rate Transition5/1
  [w] -> MATLAB Function/3(w)
  Bus Element In31/1 -> Mux1/1
  [q] -> Calc_Fx_Gx/2(q)
  [p] -> Calc_Fx_Gx/1(p)
  [K_smc_D] -> MATLAB Function3/6(kd)
  [Hx] -> MATLAB Function2/1(Hx)
  [integral_e] -> MATLAB Function3/3(integral_e)
  Calc_Fx_Gx/1(fx) -> [fx], Bus Element Out13/1
  Mux1/1 -> Rate Transition2/1
  MATLAB Function/1(H) -> Bus Element Out11/1, [Hx]
  Bus Element In25/1 -> Rate Transition1/1
  [K_REACH_P] -> MATLAB Function4/3(kp)
  [e] -> MATLAB Function3/1(e)
  [omega_phi] -> MATLAB Function1/1(omega)
  [phi] -> Omega_phi/1(phi)
  [fx] -> MATLAB Function/4(fx)
  Rate Transition3/1 -> Bus Element Out5/1
  MATLAB Function3/1(s) -> Bus Element Out10/1, MATLAB Function4/1(s)
  Bus Element In29/1 -> Mux1/3
  Demux1/3 -> [r]
  [K_smc_P] -> MATLAB Function3/4(kp)
  Demux1/2 -> [q]
  [K_smc_I] -> MATLAB Function3/5(ki)
  Discrete Derivative/1 -> Discrete Derivative1/1, Bus Element Out22/1, [phi_cmd_dot]
  Demux/3 -> [phi]
  [e] -> MATLAB Function/7(e)
  [G1x] -> MATLAB Function2/2(G1x)
  Bus Element In26/1 -> Mux/1
  Mux/1 -> Demux1/1
  [K_smc_D] -> MATLAB Function1/3(kd)
  BusElementIn2/1 -> Rate Transition6/1
  BusElementIn/1 -> Rate Transition4/1
  Demux/1 -> [psi]
  MATLAB Function2/2(G1_inv) -> Bus Element Out12/1
  Bus Element In1/1 -> Compare To Constant1/1, Compare To Constant/1
  Compare To Constant/1 -> XOR/2
  Bus Element In36/1 -> XOR/1
  BusElementIn5/1 -> Rate Transition9/1
  BusElementIn6/1 -> Rate Transition10/1
  BusElementIn7/1 -> Rate Transition11/1
  [I_XX] -> Calc_Fx_Gx/4(Ixx)
  [I_YY] -> Calc_Fx_Gx/5(Iyy)
  [I_ZZ] -> Calc_Fx_Gx/6(Izz)
  [Epsilon] -> MATLAB Function4/4(eps)
  BusElementIn8/1 -> Rate Transition12/1
  Discrete Varying Lowpass/1 -> Bus Element Out21/1, [phi_cmd], Discrete Derivative/1
  [phi_cmd] -> Subtract/1
  BusElementIn9/1 -> Gain/1
  MATLAB Function4/1(ST_R) -> Bus Element Out1/1, Switch/1
  MATLAB Function4/3(wdot) -> Discrete-Time Integrator/1
  Discrete-Time Integrator/1 -> MATLAB Function4/7(w)
  BusElementIn10/1 -> Rate Transition13/1
  BusElementIn11/1 -> Rate Transition14/1
  [lambda] -> MATLAB Function4/5(lamda)
  [eta] -> MATLAB Function4/6(eta)
  XOR/1 -> Rate Transition15/1
  [SMC_RESET] -> Discrete PID Controller2/2
  [SMC_RESET] -> Discrete-Time Integrator/2
  Compare To Constant1/1 -> Rate Transition16/1, XOR/3
  [ST_SMC_ON] -> Switch/2
  Switch/1 -> MATLAB Function2/3(R)
  Rate Transition2/1 -> Demux/1
  Rate Transition1/1 -> [des_roll]
  Rate Transition4/1 -> [K_smc_P]
  Rate Transition5/1 -> [K_smc_I]
  Rate Transition6/1 -> [K_smc_D]
  Rate Transition7/1 -> [K_REACH_S]
  Rate Transition8/1 -> [K_REACH_P]
  Rate Transition9/1 -> [I_XX]
  Rate Transition10/1 -> [I_YY]
  Rate Transition11/1 -> [I_ZZ]
  Rate Transition12/1 -> [Epsilon]
  Rate Transition13/1 -> [lambda]
  Rate Transition14/1 -> [eta]
  Rate Transition15/1 -> [SMC_RESET]
  Rate Transition16/1 -> [ST_SMC_ON]
  Gain/1 -> Rate Transition17/1
  Rate Transition17/1 -> [LPF_Cutoff]
  [LPF_Cutoff] -> Discrete Varying Lowpass/2
